simulink model "nuovo_TRACKING"  (R2024b)
settings: Solver=ode4  StartTime=0.0  StopTime=T_SIM  FixedStep=T_s  RelTol=1e-3
values from neighbouring files (symbols this model uses):
  b = 0.05    [new_traj_tracking_script.m]    (also in traj_tracking_script.m)
  control_par = [k1, k2,b]    [new_traj_tracking_script.m]    (also in traj_tracking_script.m)
  controller_index = 1    [new_traj_tracking_script.m]    (also in traj_tracking_script.m = 3)
  d = d_actual    (= 0.1604)    [new_traj_tracking_script.m]    (also in traj_tracking_script.m)
  D = diag([0.8e-3, 0.8e-3, 5e-3, 0.0175/6, 0.0175/6, 0.0175/6*T_s, 0.0175/6*T_s].^2)    [new_traj_tracking_script.m]    (also in traj_tracking_script.m = diag([1.5e-3, 1.5e-3, 1e-2, 0.0175/6, 0.0175/6, 0.0175/6*T_s)
  d_actual = 0.16040    (= 0.1604)    [new_traj_tracking_script.m]    (also in traj_tracking_script.m)
  H_enc = [0, 0, 0, 1, 0, 0, 0 ... (first row only)    [new_traj_tracking_script.m]    (also in traj_tracking_script.m)
  H_gyro = [0, 0, 0, 0, 0, -r_actual/d_actual, r_actual/d_actual]    [new_traj_tracking_script.m]    (also in traj_tracking_script.m)
  H_motion_cap = [1, 0, 0, 0, 0, 0, 0 ... (first row only)    [new_traj_tracking_script.m]    (also in traj_tracking_script.m)
  omega_M = 10    [new_traj_tracking_script.m]    (also in traj_tracking_script.m)
  P_INIT_EKF = diag([0.001, 0.001, 0.0175/6, 0.0175/6, 0.0175/6, 0.0175/6*T_s, 0.0175/6*T_s].^2)    [new_traj_tracking_script.m]    (also in traj_tracking_script.m)
  p_loss = sim_output.p_loss.signals.values(1)    [Lab2_save_data.m]    (also in new_traj_tracking_script.m = p_loss_values(i); traj_tracking_script.m = p_loss_values(i))
  PHI_INIT = [0;0]    [new_traj_tracking_script.m]    (also in traj_tracking_script.m)
  Q_INIT = [-0.4; -0.5; pi/2]    [new_traj_tracking_script.m]    (also in traj_tracking_script.m)
  Q_INIT_LOC = Q_INIT    [new_traj_tracking_script.m]    (also in traj_tracking_script.m)
  r = r_actual    (= 0.03293)    [new_traj_tracking_script.m]    (also in traj_tracking_script.m)
  R_3 = diag(([sigma_motion_capture, sigma_motion_capture, sigma_motion_capture,               sigma_enc, sigma_enc, sigma_imu]).^2)    [new_traj_tracking_script.m]    (also in traj_tracking_script.m)
  r_actual = 0.03293    [new_traj_tracking_script.m]    (also in traj_tracking_script.m)
  T_s = (sim_output.tout(end)-sim_output.tout(1))/(length(sim_output.tout)-1)    [Lab2_save_data.m]    (also in new_traj_tracking_script.m = 0.04; traj_tracking_script.m = 0.04)
  T_trj = 15    [new_traj_tracking_script.m]    (also in traj_tracking_script.m)
  trj_index = 2    [new_traj_tracking_script.m]    (also in traj_tracking_script.m)
  Z_INIT_EKF = [Q_INIT; 0; 0; 0; 0]    [new_traj_tracking_script.m]    (also in traj_tracking_script.m)
undefined symbols (not defined in the file or in its folder): X, Y
libraries: robotlib x6, sharedtransform x1
(part 2 of 2)

== matlab function nuovo_TRACKING/Planning/Trajectory Planning ==
  data: t input; q_d output; dq_d output; u_DF output; trj_index parameter; T_trj parameter
function [q_d, dq_d, u_DF] = get_trj(t, trj_index, T_trj)
if trj_index == 1
    % line
    vel = 1/T_trj;
    q_d = [0; vel*t; pi/2];
    dq_d = [0; vel; 0];
    u_DF = [vel; 0];
elseif trj_index == 2
    % circle
    r = 0.5;
    omega = 2*pi/T_trj;
    theta_prime = omega*t;
    q_d = [r*cos(theta_prime); r*sin(theta_prime); theta_prime + pi/2];
    dq_d = [-omega*r*sin(theta_prime); omega*r*cos(theta_prime); omega];
    u_DF = [omega*r; omega];
elseif trj_index == 3
    %  square
    T_cycle = mod(t, T_trj);
    side_length = 1;
    vel = side_length/(T_trj/4);
    if T_cycle<=T_trj/4
        t_side = T_cycle;
        q_d = [0;  t_side*vel; pi/2];
        dq_d = [0;vel;0];
        u_DF = [vel; 0];
    elseif T_cycle <=T_trj/2
        t_side = T_cycle - T_trj/4;
        q_d = [-vel*t_side; side_length ;pi];
        dq_d = [-vel;0;0];
        u_DF = [vel;0];
    elseif T_cycle <= 3*T_trj/4
        t_side = T_cycle - T_trj/2;
        q_d = [-side_length; side_length-vel*t_side; -pi/2];
        dq_d = [0;-vel;0];
        u_DF = [vel;0];
    else
        t_side = T_cycle - 3*T_trj/4;
        q_d = [-side_length + vel*t_side; 0; 0];
        dq_d = [vel;0;0];
        u_DF = [vel;0];
    end
elseif trj_index == 4
    % 8-shape
    R = 0.4;
    omega = 2*pi/T_trj;
    x_d = R*sin(2*omega*t);
    dx_d = R*2*omega*cos(2*omega*t);
    ddx_d = -R*4*omega.^2*sin(2*omega*t);
    y_d = R*sin(omega*t);
    dy_d = R*omega*cos(omega*t);
    ddy_d = -R*omega.^2*sin(omega*t);
    theta_d = atan2(dy_d, dx_d);
    dtheta_d = (dx_d*ddy_d -  dy_d*ddx_d)/(dx_d.^2+dy_d.^2);
    q_d = [x_d;y_d;theta_d];
    dq_d = [dx_d;dy_d;dtheta_d];
    u_DF = [sqrt(dx_d.^2 + dy_d.^2);dtheta_d];


elseif trj_index == 5
    % S cartesian traj
    
    %% --- Parametri traiettoria
    Ta = 1;
    Tc = 10;
    qi = [-0.5; -0.5; pi/2];
    qf = [ 0.5;  0.5; pi/2];
    ki = 4;
    kf = 4;
    
    %% --- Time Law Trapezoidale (scalare in t) ---
    vc = 1 / (Ta + Tc);
    a  = vc / Ta;
    T_end = 2*Ta + Tc;
    
    if t < Ta
        % Fase 1: accelerazione
        s_dot = a * t;
        s     = 0.5 * a * t^2;
    elseif t < (Ta + Tc)
        % Fase 2: velocità costante
        s_dot = vc;
        s     = 0.5 * a * Ta^2 + vc * (t - Ta);
    elseif t < T_end
        % Fase 3: decelerazione
        dt3   = t - Ta - Tc;
        s_dot = vc - a * dt3;
        s     = 0.5*a*Ta^2 + vc*Tc + vc*dt3 - 0.5*a*dt3^2;
    else
        % Fase 4: fine traiettoria
        s_dot = 0;
        s     = 1;
    end
    
    %% --- Polinomi Cubici ---
    xi = qi(1); yi = qi(2); thetai = qi(3);
    xf = qf(1); yf = qf(2); thetaf = qf(3);
    
    coeff_a = [xf,  xi,  kf*cos(thetaf) - 3*xf,  ki*cos(thetai) + 3*xi];
    coeff_b = [yf,  yi,  kf*sin(thetaf) - 3*yf,  ki*sin(thetai) + 3*yi];
    
    % Posizione geometrica
    x_s = coeff_a(1)*s^3 - coeff_a(2)*(s^3-3*s^2+3*s-1) ...
        + coeff_a(3)*(s^3-s^2) + coeff_a(4)*(s^3-2*s^2+s);
    y_s = coeff_b(1)*s^3 - coeff_b(2)*(s^3-3*s^2+3*s-1) ...
        + coeff_b(3)*(s^3-s^2) + coeff_b(4)*(s^3-2*s^2+s);
    
    % Prima derivata rispetto a s
    x_ds = 3*coeff_a(1)*s^2 - coeff_a(2)*(3*s^2-6*s+3) ...
         + coeff_a(3)*(3*s^2-2*s) + coeff_a(4)*(3*s^2-4*s+1);
    y_ds = 3*coeff_b(1)*s^2 - coeff_b(2)*(3*s^2-6*s+3) ...
         + coeff_b(3)*(3*s^2-2*s) + coeff_b(4)*(3*s^2-4*s+1);
    
    % Seconda derivata rispetto a s
    x_dds = 6*coeff_a(1)*s - coeff_a(2)*(6*s-6) + coeff_a(3)*(6*s-2) + coeff_a(4)*(6*s-4);
    y_dds = 6*coeff_b(1)*s - coeff_b(2)*(6*s-6) + coeff_b(3)*(6*s-2) + coeff_b(4)*(6*s-4);
    
    %% --- Input geometrici ---
    v_tilde     = sqrt(x_ds^2 + y_ds^2);
    omega_tilde = (x_ds * y_dds - y_ds * x_dds) / (x_ds^2 + y_ds^2);
    
    %% --- Input reali (feedforward) ---
    v = v_tilde * s_dot;
    w = omega_tilde * s_dot;

    u_DF = [v;w];
    
    %% --- Stato desiderato q_d = [x; y; theta] ---
    theta_d = atan2(y_ds, x_ds);   % orientamento tangente alla curva
    q_d  = [x_s; y_s; theta_d];
    
    %% --- Velocità desiderata dq_d = [dx; dy; dtheta] ---
    % Per un unicycle: dx = v*cos(theta), dy = v*sin(theta), dtheta = w
    dq_d = [v * cos(theta_d);
            v * sin(theta_d);
            w];
else
    q_d = [0;0;0];
    dq_d = [0;0;0];
    u_DF = [0;0];
end

== matlab function nuovo_TRACKING/Localizzazione EKF/MATLAB Function2 ==
  data: P_filt input; P_new output; z_filt input; z_new output; u input; y_new input; D parameter; T_s parameter; r_actual parameter; d_actual parameter; H_enc parameter; H_gyro parameter; H_motion_cap parameter; R_3 parameter; q_EKF output
function [P_new, z_new, q_EKF] = EKF_filtering(P_filt, z_filt, u, y_new, D, T_s, r_actual, d_actual, H_enc, H_gyro, H_motion_cap, R_3)

    % Def state z_filt: [xk , yk , thetak , delta_phi_L_km1 , delta_phi_R_km1 , wLk , wRk ]

    r = r_actual;
    d = d_actual;
        
    % Extraction variables
    x_k = z_filt(1);
    y_k = z_filt(2);
    theta_k = z_filt(3);
    delta_phi_L_km1 = z_filt(4);
    delta_phi_R_km1 = z_filt(5); 
    wL_k = z_filt(6);               % estimate wheels velocities
    wR_k = z_filt(7);
    
    uL_k = u(1);                    % actual wheels velocities (from command input v,w)
    uR_k = u(2);

    % ----------------------

    % PREDICT STEP
    v_k = (r/2) * (wL_k + wR_k);
    omega_k = (r/d) * (wR_k - wL_k);
    theta_mean = theta_k + (omega_k * T_s) / 2;
        
    % State Prediction (approximation with RK2)
    x_kp1 = x_k + v_k * T_s * cos(theta_mean);
    y_kp1 = y_k + v_k * T_s * sin(theta_mean);
    theta_kp1 = theta_k + omega_k * T_s;
    
    delta_phi_L_k = wL_k * T_s;
    delta_phi_R_k = wR_k * T_s;
    
    wL_kp1 = uL_k; 
    wR_kp1 = uR_k;
    
    z_hat = [x_kp1; y_kp1; theta_kp1; delta_phi_L_k; delta_phi_R_k; wL_kp1; wR_kp1];
    
    % F derivation
    F = zeros(7,7);
    
    F(1,1) = 1;
    F(1, 3) = -T_s * v_k * sin(theta_mean);
    F(1, 6) = (T_s * r / 2) * cos(theta_mean) - v_k * T_s * sin(theta_mean) * (-T_s * r / (2 * d));
    F(1, 7) = (T_s * r / 2) * cos(theta_mean) - v_k * T_s * sin(theta_mean) * (T_s * r / (2 * d));
    
    F(2,2) = 1;
    F(2, 3) = v_k * T_s * cos(theta_mean);
    F(2, 6) = (T_s * r / 2) * sin(theta_mean) + v_k * T_s * cos(theta_mean) * (-T_s * r / (2 * d));
    F(2, 7) = (T_s * r / 2) * sin(theta_mean) + v_k * T_s * cos(theta_mean) * (T_s * r / (2 * d));

    F(3,3) = 1;
    F(3, 6) = -T_s * r / d;
    F(3, 7) = T_s * r / d;

    F(4, 6) = T_s;
    F(5, 7) = T_s;
    
    % Covariance Prediction
    P_hat = F * P_filt * F' + D;
    
    % ----------------------

    % UPDATE STEP
    % H and R will depend on the measurement data y_new and Test_case

    % enc_values (delta_phi)
    % IMU_values (w_gyro)
    % Motion_capture (state q)

    % y_new = [x; y; theta; delta_phi_L; delta_phi_R; omega_gyro]

    %% OBSERVATION MATRIX H ALWAYS FULL (6X7) AND ALSO Y_NEW (6X1) 
    H_full = [H_motion_cap; H_enc; H_gyro];
    y_meas = y_new; 


    % Start with full matrix R_3 
    R_current = R_3;
    INFINITY_VAR = 1e9; % Infinite var to put down the Kalman gain
    
    % IMU not available
    R_current(6,6) = INFINITY_VAR; 

    % TEST 3: all active, possibile data loss
    if any(isnan(y_new(1:3)))   
        y_meas(1:3) = 0;    % force to zero just for completness
        R_current(1,1) = INFINITY_VAR; 
        R_current(2,2) = INFINITY_VAR; 
        R_current(3,3) = INFINITY_VAR;
    end
    
    % Innovation e_pred
    y_hat = H_full * z_hat;
    e_kp1 = y_meas - y_hat;
    
    % Kalman Gain K_pred
    K = P_hat * H_full' / (H_full * P_hat * H_full' + R_current);   
    
    % State and Covariance Update
    z_new = z_hat + K * e_kp1;
    P_new = P_hat - K * H_full * P_hat;

    q_EKF = z_new(1:3);


end

== matlab function nuovo_TRACKING/Norm cartesian error ==
  data: u input; y output
function y = fcn(u)

y = sqrt(sum(u(1:2).^2));
